simulink library "pwm_sig_converters"  (R2018b)
settings: Solver=VariableStepAuto  StartTime=0.0  StopTime=10.0  RelTol=1e-3
settings Model: Creator=Robert  LastModifiedBy=Robert

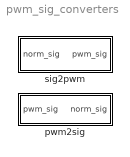
== system pwm_sig_converters ==
  pwm2sig : Subsystem
  sig2pwm : Subsystem

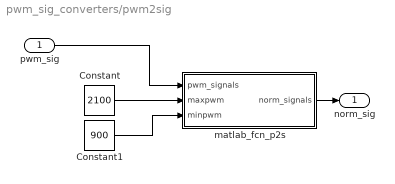
== system pwm_sig_converters/pwm2sig ==
  pwm_sig : Inport
  Constant : Constant  Value=2100  OutDataTypeStr=uint16
  Constant1 : Constant  Value=900  OutDataTypeStr=uint16
  matlab_fcn_p2s : MATLAB Function  TreatAsAtomicUnit=on
  norm_sig : Outport
  wires:
  matlab_fcn_p2s/1(norm_signals) -> norm_sig/1
  Constant1/1 -> matlab_fcn_p2s/3(minpwm)
  Constant/1 -> matlab_fcn_p2s/2(maxpwm)
  pwm_sig/1 -> matlab_fcn_p2s/1(pwm_signals)

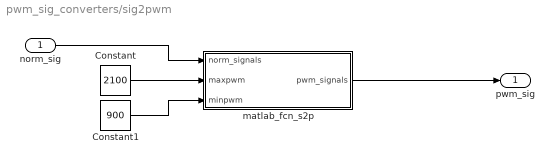
== system pwm_sig_converters/sig2pwm ==
  norm_sig : Inport
  Constant : Constant  Value=2100  OutDataTypeStr=uint16
  Constant1 : Constant  Value=900  OutDataTypeStr=uint16
  matlab_fcn_s2p : MATLAB Function  TreatAsAtomicUnit=on
  pwm_sig : Outport
  wires:
  Constant/1 -> matlab_fcn_s2p/2(maxpwm)
  matlab_fcn_s2p/1(pwm_signals) -> pwm_sig/1
  Constant1/1 -> matlab_fcn_s2p/3(minpwm)
  norm_sig/1 -> matlab_fcn_s2p/1(norm_signals)

== matlab function pwm_sig_converters/pwm2sig/matlab_fcn_p2s ==
  data: pwm_signals input uint16; norm_signals output single; maxpwm input uint16; minpwm input uint16
function norm_signals = pwm2signal(pwm_signals, maxpwm, minpwm)

y = single(pwm_signals);

top =   uint16(maxpwm);
bot =   uint16(minpwm);
mid =   uint16((single(top)+single(bot))/2);
range = uint16( (single(top)-single(bot))/2 );

y = (y - single(mid))./(single(range)); 

norm_signals = y;

== matlab function pwm_sig_converters/sig2pwm/matlab_fcn_s2p ==
  data: norm_signals input single; pwm_signals output uint16; maxpwm input uint16; minpwm input uint16
function pwm_signals = signal2pwm(norm_signals, maxpwm, minpwm)

pwm_signals = uint16(zeros(size(norm_signals))); % y is hard set to uint16


top =   uint16(maxpwm);
bot =   uint16(minpwm);
mid =   uint16((single(top)+single(bot))/2);
range = uint16( (single(top)-single(bot))/2 );

% Range is ~1000-2000, ie +-500, but in is +-1
norm_signals = norm_signals.*single(range) + single(mid);
pwm_signals = uint16(norm_signals);
